simulink model "SC_Model_Sim_w3_final"  (R2023b)
settings: Solver=ode45  StartTime=0.0  StopTime=inf  FixedStep=0.001  RelTol=1e-3
values from neighbouring files (symbols this model uses):
  invJ = inv(J)    [SC_Model_Par.m]
  J = [J_11  0   0 ... (first row only)    [SC_Model_Par.m]
  J_w = wheel_momentum_max/wheel_speed_max    (= 0.000713699296376)    [SC_Model_Par.m]
  k_d = 0.2    [SC_Model_Par.m]
  k_p = 0.0041    [SC_Model_Par.m]
  mu_0 = 1.25663706212e-6    (= 1.25663706212e-06)    [SC_Model_Par.m]
  q_0 = dcm2quat(DCM_0)    [SC_Model_Par.m]
  R_E = 6371.2e3    (= 6371200)    [SC_Model_Par.m]
  wheel_momentum_max = 0.05    [SC_Model_Par.m]
  wheel_torque_max = 20e-3    (= 0.02)    [SC_Model_Par.m]
undefined symbols (not defined in the file or in its folder): IAU, juliandate, M, phi_n, theta_n, WMM2020
libraries: sharedtransform x3, vrlib x3, sharedutil x2, simulink x1, aerolibtransform2 x1, aerolibgravity2 x1
settings Model: SimulationMode=accelerator  Creator=andry  LastModifiedBy=Thien
settings SolverCC: ZeroCrossAlgorithm=Adaptive
settings DebuggingCC: MaskedZcDiagnostic=none  IgnoredZcDiagnostic=none  UnconnectedInputMsg=warning  UnconnectedOutputMsg=warning  UnconnectedLineMsg=warning
settings ModelReferenceCC: EnableRefExpFcnMdlSchedulingChecks=on
settings RTWCC: DLArmComputeVersion=19.05

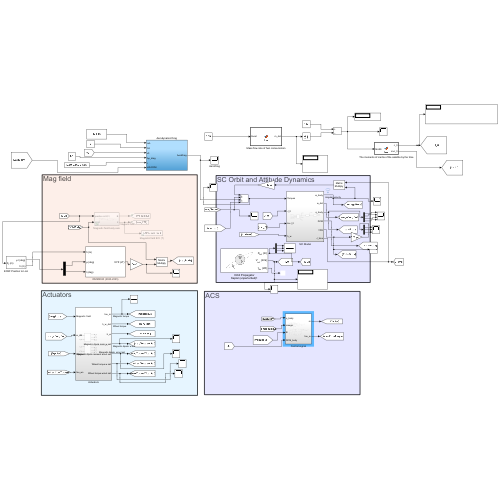
[thumbnail: Simulink's stored preview of the top-level diagram]
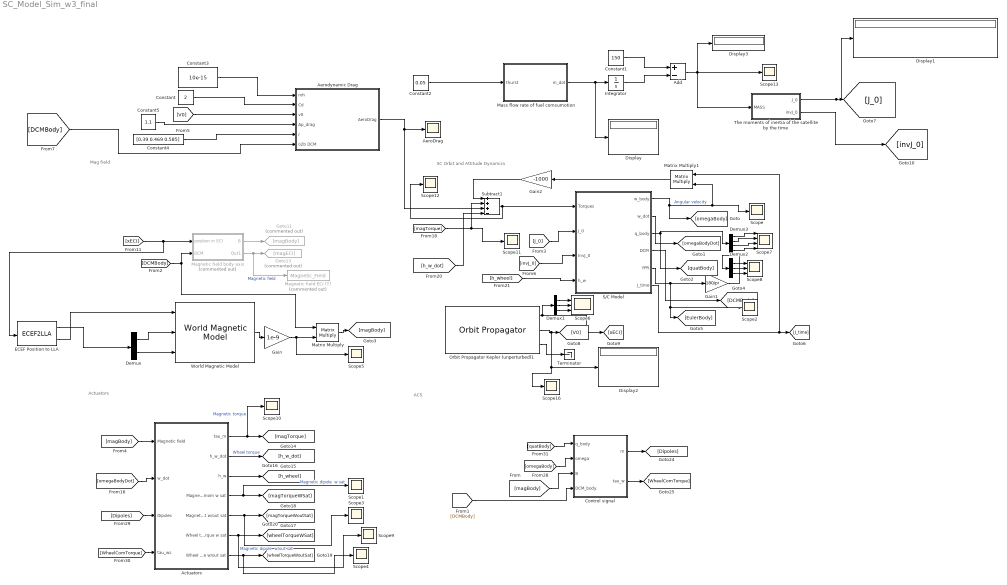
== system SC_Model_Sim_w3_final ==
  note: ACS
  note: Actuators
  note: SC Orbit and Attitude Dynamics
  note: Mag field
  Actuators : Subsystem
  Add : Sum  Inputs=+-
  AeroDrag : Scope
  Aerodynamic Drag : Subsystem
  Constant : Constant  Value=2
  Constant1 : Constant  Value=150  SampleTime=0
  Constant2 : Constant  Value=0.05  VectorParams1D=off
  Constant3 : Constant  Value=10e-15
  Constant4 : Constant  Value=[0.39 0.469 0.585]
  Constant5 : Constant  Value=1.1
  Control signal : Subsystem
  Demux : Demux  Outputs=2
  Demux1 : Demux  Outputs=3
  Demux2 : Demux  Outputs=3
  Demux3 : Demux
  Display{,1..3} (4 alike) : Display
      Display settings: Decimation=2
      Display1 settings: Decimation=3
  ECEF Position to LLA : ECEF2LLA
  Gain : Gain  Gain=1e-9
  Gain1 : Gain  Gain=180/pi
  Gain2 : Gain  Gain=-1000
  Goto11 : Goto  Commented=on  GotoTag=magBody
  Goto13 : Goto  Commented=on  GotoTag=magECI
  Integrator : Integrator  InitialCondition=35e-1000000  LimitOutput=on  UpperSaturationLimit=10  LowerSaturationLimit=0
  Magnetic field ECI (T) : ToWorkspace  Commented=on  VariableName=Magnetic_Field  SaveFormat=Timeseries  SampleTime=-1
  Magnetic field body axis : Subsystem  Commented=on
  Mass flow rate of fuel comsumotion : MATLAB Function  TreatAsAtomicUnit=on
  Matrix Multiply : Product  Multiplication=Matrix(*)
  Matrix Multiply1 : Product  Multiplication=Matrix(*)
  Orbit Propagator Kepler (unperturbed)1 : OrbitPropagator  outportFrame=Fixed-frame  startDate=juliandate(2022, 4, 25, 12, 0, 0)  semiMajorAxis=sma  eccentricity=ecc  inclination=orb_i  raan=RAAN  argPeriapsis=arg_per  trueAnomaly=0*pi/180  inertialPosition=[3649700.0 3308200.0 -4676600.0]  inertialVelocity=[-2750.8 6666.4 2573.4]  fixedPosition=[-4142689.0 -2676864.7 -4669861.6]  fixedVelocity=[1452.7 -6720.7 2568.1]  gravityModel=None  customR=3396200  customMu=4.305e13  customJ2=1.0826269e-03  customOmega=4.06125949e-3  useEOPs=off  angleUnits=Radians
  S/C Model : Subsystem
  Scope{,1..5,9..13,16} (12 alike) : Scope
  Scope6 : Scope  NumInputPorts=3
  Scope7 : Scope  NumInputPorts=4
  Scope8 : Scope  NumInputPorts=3
  Subtract1 : Sum  Inputs=+++-
  Terminator : Terminator
  The moments of inertia of the satellite by the time : MATLAB Function  TreatAsAtomicUnit=on
  World Magnetic Model : aerolibgravity2/World Magnetic Model  model=WMM2020 (2020-2025)  customFile='WMM2020.COF'  units=Metric (MKS)  time_in=off  month=April  day=25  year=2022  action=Error  h_out=off  dec_out=off  inc_out=off  ti_out=off
  wires:
  S/C Model/1(w_body) -> [omegaBody], Matrix Multiply1/2, Scope/1  "Angular velocity"
  S/C Model/2(w_dot) -> [omegaBodyDot]
  [DCMBody] -> Magnetic field body axis/2(DCM), Matrix Multiply/1
  S/C Model/5(YPR) -> [EulerBody], Scope2/1, Gain1/1
  [xECI] -> Magnetic field body axis/1(position in ECI), ECEF Position to LLA/1
  Orbit Propagator Kepler (unperturbed)1/2 -> Scope16/1, Display2/1, [V0]
  Magnetic field body axis/1(B) -> Goto11/1
  Magnetic field body axis/2(Out1) -> Magnetic field ECI (T)/1, Goto13/1  "Magnetic field"
  Actuators/1(tau_m) -> Scope10/1, [magTorque]  "Magnetic torque"
  Actuators/2(h_w_dot) -> [h_w_dot]  "Wheel torque"
  Actuators/3(h_w) -> [h_wheel]
  [h_wheel] -> S/C Model/4(h_w)
  Actuators/5(Magnetic dipole moment w/out sat) -> Scope3/1, [magTorqueWoutSat]  "Magnetic dipole  w/out sat"
  Actuators/4(Magnetic dipole mom w sat) -> Scope1/1, [magTorqueWSat]  "Magnetic dipole  w sat"
  Actuators/7(Wheel torque w/out sat) -> Scope4/1, [wheelTorqueWoutSat]
  Actuators/6(Wheel torque w sat) -> Scope9/1, [wheelTorqueWSat]
  [magBody] -> Actuators/1(Magnetic field)
  [omegaBodyDot] -> Actuators/2(w_dot)
  Control signal/1(m) -> [Dipoles]
  Control signal/2(tau_w) -> [WheelComTorque]
  [Dipoles] -> Actuators/3(Dipoles)
  [WheelComTorque] -> Actuators/4(tau_ws)
  Orbit Propagator Kepler (unperturbed)1/3 -> Terminator/1
  [quatBody] -> Control signal/1(q_body)
  [omegaBody] -> Control signal/2(omega)
  [magBody] -> Control signal/3(B)
  ECEF Position to LLA/2 -> World Magnetic Model/1
  ECEF Position to LLA/1 -> Demux/1
  Demux/1 -> World Magnetic Model/2
  Demux/2 -> World Magnetic Model/3
  World Magnetic Model/1 -> Gain/1
  Matrix Multiply/1 -> [magBody]
  Demux1/1 -> Scope6/1
  Demux1/2 -> Scope6/2
  Demux1/3 -> Scope6/3
  Orbit Propagator Kepler (unperturbed)1/1 -> Demux1/1, [xECI]
  Gain/1 -> Scope5/1, Matrix Multiply/2
  S/C Model/3(q_body) -> Demux3/1, [quatBody]
  Demux2/1 -> Scope8/1
  Demux2/2 -> Scope8/2
  Demux2/3 -> Scope8/3
  Gain1/1 -> Demux2/1
  Demux3/1 -> Scope7/1
  Demux3/2 -> Scope7/2
  Demux3/3 -> Scope7/3
  Demux3/4 -> Scope7/4
  [magTorque] -> Scope11/1, Subtract1/2
  Gain2/1 -> Subtract1/1
  Subtract1/1 -> Scope12/1, S/C Model/1(Torques)
  The moments of inertia of the satellite by the time/1(J_0) -> Display1/1, [J_0]
  [V0] -> Aerodynamic Drag/3(v0)
  Constant/1 -> Aerodynamic Drag/2(Cd)
  [J_0] -> S/C Model/2(J_0)
  The moments of inertia of the satellite by the time/2(invJ_0) -> [invJ_0]
  [invJ_0] -> S/C Model/3(InvJ_0)
  Matrix Multiply1/1 -> Gain2/1
  S/C Model/6(J_time) -> [J_time], Matrix Multiply1/1
  Constant2/1 -> Mass flow rate of fuel comsumotion/1(thurst)
  Mass flow rate of fuel comsumotion/1(m_dot) -> Display/1, Integrator/1
  Add/1 -> The moments of inertia of the satellite by the time/1(MASS), Scope13/1, Display3/1
  Integrator/1 -> Add/2
  Constant1/1 -> Add/1
  [DCMBody] -> Control signal/4(DCM_body)
  Constant3/1 -> Aerodynamic Drag/1(roh)
  Constant4/1 -> Aerodynamic Drag/5(r)
  Constant5/1 -> Aerodynamic Drag/4(Ap_drag)
  S/C Model/4(DCM) -> [DCMBody]
  [h_w_dot] -> Subtract1/4
  Aerodynamic Drag/1(AeroDrag) -> Subtract1/3, AeroDrag/1
  [DCMBody] -> Aerodynamic Drag/6(o2b DCM)

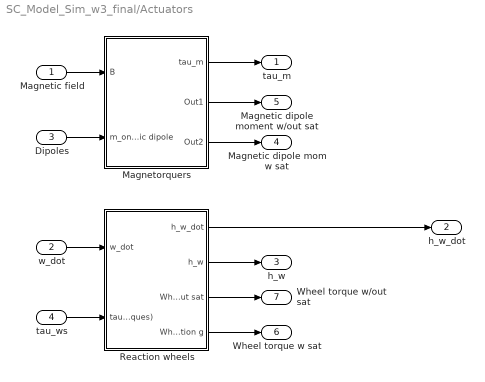
== system SC_Model_Sim_w3_final/Actuators ==
  Magnetic field : Inport
  w_dot : Inport  Port=2
  Dipoles : Inport  Port=3
  tau_ws : Inport  Port=4
  Magnetorquers : Subsystem
  Reaction wheels : Subsystem
  tau_m : Outport
  h_w_dot : Outport  Port=2
  h_w : Outport  Port=3
  Magnetic dipole mom w sat : Outport  Port=4
  Magnetic dipole moment w/out sat : Outport  Port=5
  Wheel torque w sat : Outport  Port=6
  Wheel torque w/out sat : Outport  Port=7
  wires:
  w_dot/1 -> Reaction wheels/1(w_dot)
  Reaction wheels/1(h_w_dot) -> h_w_dot/1
  Reaction wheels/2(h_w) -> h_w/1
  Magnetorquers/2(Out1) -> Magnetic dipole moment w/out sat/1
  Magnetorquers/3(Out2) -> Magnetic dipole mom w sat/1
  Reaction wheels/4(Wheel torque w saturation g) -> Wheel torque w sat/1
  Reaction wheels/3(Wheel torque w/out sat) -> Wheel torque w/out sat/1
  Dipoles/1 -> Magnetorquers/2(m_onboard magnetic dipole)
  Magnetic field/1 -> Magnetorquers/1(B)
  tau_ws/1 -> Reaction wheels/2(tau_w (control torques))
  Magnetorquers/1(tau_m) -> tau_m/1

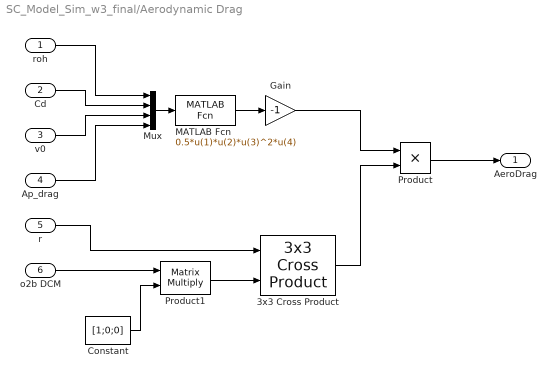
== system SC_Model_Sim_w3_final/Aerodynamic Drag ==
  roh : Inport
  Cd : Inport  Port=2
  v0 : Inport  Port=3
  Ap_drag : Inport  Port=4
  r : Inport  Port=5
  o2b DCM : Inport  Port=6
  3x3 Cross Product : sharedutil/3x3 Cross Product  aMode=aMode
      settings: LibrarySourceBlock=aerolibutil/3x3 Cross Product
  Constant : Constant  Value=[1;0;0]
  Gain : Gain  Gain=-1
  MATLAB Fcn : MATLABFcn  MATLABFcn=0.5*u(1)*u(2)*u(3)^2*u(4)
  Mux : Mux
  Product : Product  RndMeth=Zero
  Product1 : Product  Multiplication=Matrix(*)  RndMeth=Zero
  AeroDrag : Outport
  wires:
  Mux/1 -> MATLAB Fcn/1
  roh/1 -> Mux/1
  Cd/1 -> Mux/2
  v0/1 -> Mux/3
  Ap_drag/1 -> Mux/4
  Constant/1 -> Product1/2
  o2b DCM/1 -> Product1/1
  Product1/1 -> 3x3 Cross Product/2
  r/1 -> 3x3 Cross Product/1
  MATLAB Fcn/1 -> Gain/1
  Gain/1 -> Product/1
  3x3 Cross Product/1 -> Product/2
  Product/1 -> AeroDrag/1

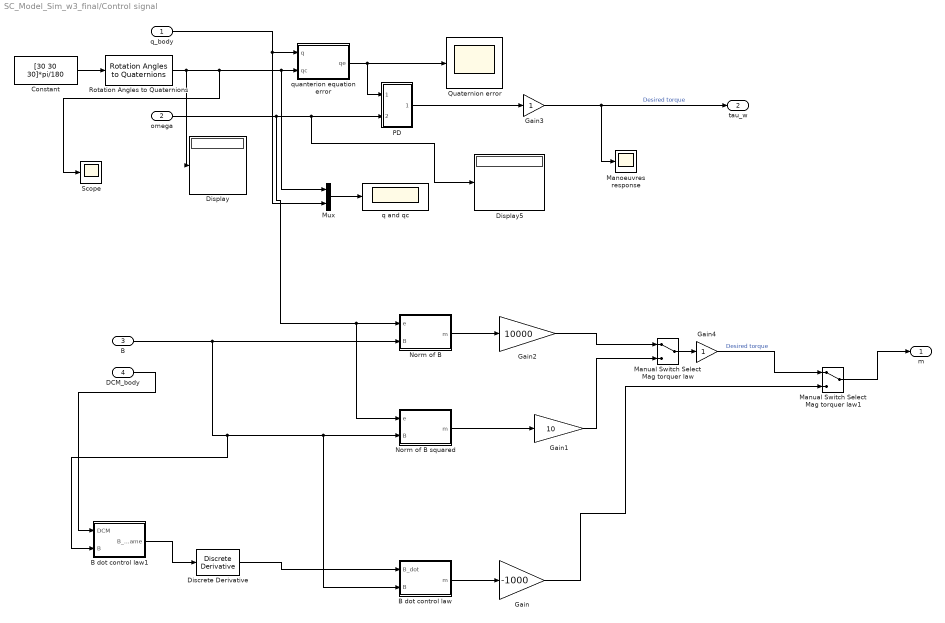
== system SC_Model_Sim_w3_final/Control signal ==
  q_body : Inport
  omega : Inport  Port=2
  B : Inport  Port=3
  DCM_body : Inport  Port=4
  B dot control law : MATLAB Function  TreatAsAtomicUnit=on
  B dot control law1 : MATLAB Function  TreatAsAtomicUnit=on
  Constant : Constant  Value=[30 30 30]*pi/180  VectorParams1D=off
  Discrete Derivative : simulink/Discrete/Discrete Derivative  gainval=1.0  ICPrevScaledInput=0.0  OutMin=[]  OutMax=[]  OutDataType=fixdt(1, 16)  OutScaling=2^-10  DoSatur=off
  Display : Display
  Display5 : Display
  Gain : Gain  Gain=-1000
  Gain1 : Gain  Gain=10
  Gain2 : Gain  Gain=10000
  Gain3 : Gain
  Gain4 : Gain
  Manoeuvres response : Scope
  Manual Switch Select Mag torquer law : ManualSwitch
  Manual Switch Select Mag torquer law1 : ManualSwitch
  Mux : Mux  Inputs=2
  Norm of B : MATLAB Function  TreatAsAtomicUnit=on
  "Norm of B squared " : MATLAB Function  TreatAsAtomicUnit=on
  PD : Subsystem
  Quaternion error : Scope
  Rotation Angles to Quaternions : sharedtransform/Rotation Angles to Quaternions  rotationOrder=ZYX  aMode=aMode
  Scope : Scope
  q and qc : Scope
  quanterion equation error : MATLAB Function  TreatAsAtomicUnit=on
  m : Outport
  tau_w : Outport  Port=2
  wires:
  PD/1(tau) -> Gain3/1
  Gain3/1 -> tau_w/1, Manoeuvres response/1  "Desired torque"
  omega/1 -> "Norm of B squared "/1(e), Norm of B/1(e), Display5/1, PD/2(w_body)
  Manual Switch Select Mag torquer law/1 -> Gain4/1
  Norm of B/1(m) -> Gain2/1
  Gain1/1 -> Manual Switch Select Mag torquer law/2
  "Norm of B squared "/1(m) -> Gain1/1
  Constant/1 -> Rotation Angles to Quaternions/1
  quanterion equation error/1(qe) -> PD/1(q_body), Quaternion error/1
  q_body/1 -> Mux/2, quanterion equation error/1(q)
  Mux/1 -> q and qc/1
  Rotation Angles to Quaternions/1 -> Scope/1, Mux/1, quanterion equation error/2(qc), Display/1
  B/1 -> B dot control law1/2(B), B dot control law/2(B), "Norm of B squared "/2(B), Norm of B/2(B)
  Gain2/1 -> Manual Switch Select Mag torquer law/1
  B dot control law/1(m) -> Gain/1
  Gain/1 -> Manual Switch Select Mag torquer law1/2
  Discrete Derivative/1 -> B dot control law/1(B_dot)
  Gain4/1 -> Manual Switch Select Mag torquer law1/1  "Desired torque"
  Manual Switch Select Mag torquer law1/1 -> m/1
  B dot control law1/1(B_bodyframe) -> Discrete Derivative/1
  DCM_body/1 -> B dot control law1/1(DCM)

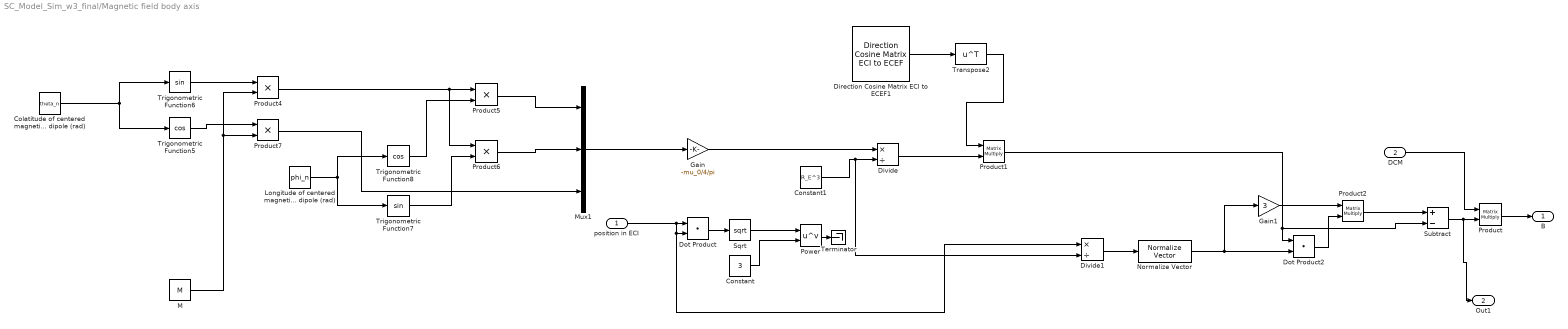
== system SC_Model_Sim_w3_final/Magnetic field body axis ==
  position in ECI : Inport
  DCM : Inport  Port=2
  Colatitude of centered magnetic dipole (rad) : Constant  Value=theta_n
  Constant : Constant  Value=3
  Constant1 : Constant  Value=R_E^3
  Direction Cosine Matrix ECI to ECEF1 : aerolibtransform2/Direction Cosine Matrix ECI to ECEF  red=IAU-2000/2006  year=2020  month=January  day=1  hour=0  min=0  sec=0  deltaT=None  errorflag=Error  extraparamflag=off
      settings: AttributesFormatString=%<red>
  Divide : Product  Inputs=*/
  Divide1 : Product  Inputs=*/
  Dot Product : DotProduct  OutDataTypeStr=Inherit: Inherit via internal rule
  Dot Product2 : DotProduct  OutDataTypeStr=Inherit: Inherit via internal rule
  Gain : Gain  Gain=-mu_0/4/pi
  Gain1 : Gain  Gain=3
  Longitude of centered magnetic dipole (rad) : Constant  Value=phi_n
  M : Constant  Value=M
  Mux1 : Mux  Inputs=3
  Normalize Vector : vrlib/Utilities/Normalize Vector  maxzero=0
  Power : Math  Operator=pow
  Product : Product  Multiplication=Matrix(*)
  Product1 : Product  Multiplication=Matrix(*)
  Product2 : Product  Multiplication=Matrix(*)
  Product{4..7} (4 alike) : Product
  Sqrt : Sqrt
  Subtract : Sum  Inputs=+-
  Terminator : Terminator
  Transpose2 : Math  Operator=transpose  SignedPower=on  RndMeth=Zero
  Trigonometric Function5 : Trigonometry  Operator=cos
  Trigonometric Function6 : Trigonometry
  Trigonometric Function7 : Trigonometry
  Trigonometric Function8 : Trigonometry  Operator=cos
  B : Outport
  Out1 : Outport  Port=2
  wires:
  Longitude of centered magnetic dipole (rad)/1 -> Trigonometric Function7/1, Trigonometric Function8/1
  Product4/1 -> Product6/1, Product5/1
  Product6/1 -> Mux1/2
  M/1 -> Product7/2, Product4/2
  Colatitude of centered magnetic dipole (rad)/1 -> Trigonometric Function5/1, Trigonometric Function6/1
  Trigonometric Function7/1 -> Product6/2
  Trigonometric Function6/1 -> Product4/1
  Product7/1 -> Mux1/3
  Trigonometric Function8/1 -> Product5/2
  Product5/1 -> Mux1/1
  Trigonometric Function5/1 -> Product7/1
  Mux1/1 -> Gain/1
  Dot Product/1 -> Sqrt/1
  Constant/1 -> Power/2
  Sqrt/1 -> Power/1
  Gain/1 -> Divide/1
  Divide/1 -> Product1/2
  Direction Cosine Matrix ECI to ECEF1/1 -> Transpose2/1
  Transpose2/1 -> Product1/1
  Subtract/1 -> Out1/1, Product/2
  Dot Product2/1 -> Product2/2
  Gain1/1 -> Product2/1
  Product2/1 -> Subtract/1
  position in ECI/1 -> Dot Product/2, Divide1/1, Dot Product/1
  Product1/1 -> Subtract/2, Dot Product2/1
  DCM/1 -> Product/1
  Product/1 -> B/1
  Constant1/1 -> Divide/2, Divide1/2
  Divide1/1 -> Normalize Vector/1
  Normalize Vector/1 -> Gain1/1, Dot Product2/2
  Power/1 -> Terminator/1

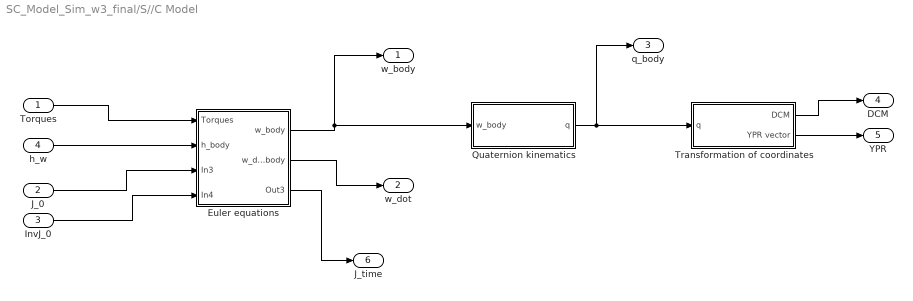
== system SC_Model_Sim_w3_final/S//C Model ==
  Torques : Inport
  J_0 : Inport  Port=2
  InvJ_0 : Inport  Port=3
  h_w : Inport  Port=4
  Euler equations : Subsystem
  Quaternion kinematics : Subsystem
  Transformation of coordinates : Subsystem
  w_body : Outport
  w_dot : Outport  Port=2
  q_body : Outport  Port=3
  DCM : Outport  Port=4
  YPR : Outport  Port=5
  J_time : Outport  Port=6
  wires:
  Quaternion kinematics/1(q) -> q_body/1, Transformation of coordinates/1(q)
  Transformation of coordinates/2(YPR vector) -> YPR/1
  Euler equations/2(w_dot_body) -> w_dot/1
  h_w/1 -> Euler equations/2(h_body)
  Transformation of coordinates/1(DCM) -> DCM/1
  Euler equations/1(w_body) -> w_body/1, Quaternion kinematics/1(w_body)
  Torques/1 -> Euler equations/1(Torques)
  J_0/1 -> Euler equations/3(In3)
  InvJ_0/1 -> Euler equations/4(In4)
  Euler equations/3(Out3) -> J_time/1

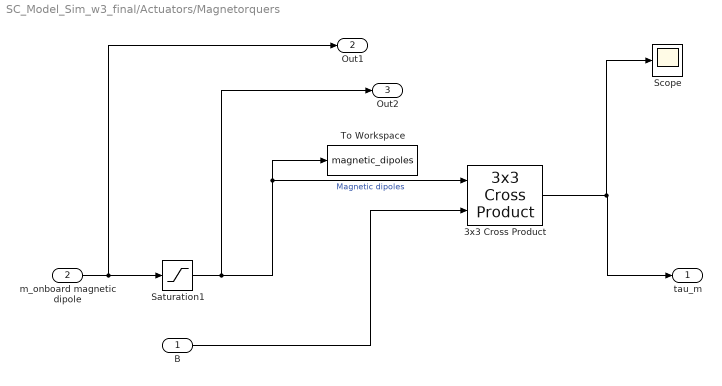
== system SC_Model_Sim_w3_final/Actuators/Magnetorquers ==
  B : Inport
  m_onboard magnetic dipole : Inport  Port=2
  3x3 Cross Product : sharedutil/3x3 Cross Product  aMode=aMode
  Saturation1 : Saturate  UpperLimit=20  LowerLimit=-20
  Scope : Scope
  To Workspace : ToWorkspace  VariableName=magnetic_dipoles  SaveFormat=Timeseries  SampleTime=-1
  tau_m : Outport
  Out1 : Outport  Port=2
  Out2 : Outport  Port=3
  wires:
  B/1 -> 3x3 Cross Product/2
  3x3 Cross Product/1 -> Scope/1, tau_m/1
  Saturation1/1 -> Out2/1, 3x3 Cross Product/1, To Workspace/1  "Magnetic dipoles"
  m_onboard magnetic dipole/1 -> Out1/1, Saturation1/1

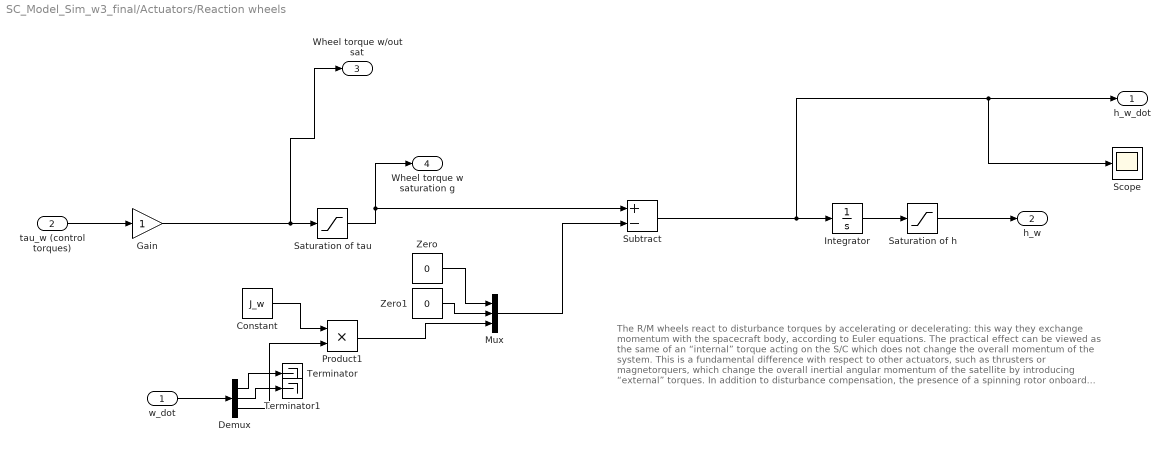
== system SC_Model_Sim_w3_final/Actuators/Reaction wheels ==
  note: The R/M wheels react to disturbance torques by accelerating or decelerating: this way they exchange momentum with the
      | spacecraft body, according to Euler equations. The practical effect can be viewed as the same of an “internal” torque acting
      | on the S/C which does not change the overall momentum of the system. This is a fundamental difference with respect to
      | other actuators, such as thrusters or magnetorquers, which change the overall inertial angular momentum of the satellite by
      | introducing “external” torques.
      | In addition to disturbance compensation, the presence of a spinning rotor onboard generates a gyroscopic stiffness
      | (i.e. storage of angular momentum) making the S/C less sensitive to the disturbance torques. Depending on which of the two
      | features above, reaction to disturbance or storage of momentum, is given the priority, a distinction is made between reaction wheels (RW)
      | or momentum wheels (MW).
      | A MW is used to keep the actuation axis almost inertially fixed by rotating at a nominal rate different
      | from zero; a control of the attitude about the rotation axis is allowed by variation of the wheel speed.
      | Conversely, RWs have zero nominal speed.
  w_dot : Inport
  tau_w (control torques) : Inport  Port=2
  Constant : Constant  Value=J_w
  Demux : Demux  Outputs=3
  Gain : Gain
  Integrator : Integrator
  Mux : Mux  Inputs=3
  Product1 : Product
  Saturation of h : Saturate  UpperLimit=wheel_momentum_max*100  LowerLimit=-wheel_momentum_max*100
  Saturation of tau : Saturate  UpperLimit=wheel_torque_max  LowerLimit=-wheel_torque_max
  Scope : Scope
  Subtract : Sum  Inputs=+-
  Terminator : Terminator
  Terminator1 : Terminator
  Zero : Constant  Value=0  OutDataTypeStr=Inherit: Inherit via back propagation
  Zero1 : Constant  Value=0  OutDataTypeStr=Inherit: Inherit via back propagation
  h_w_dot : Outport
  h_w : Outport  Port=2
  Wheel torque w/out sat : Outport  Port=3
  Wheel torque w saturation g : Outport  Port=4
  wires:
  Constant/1 -> Product1/1
  w_dot/1 -> Demux/1
  Demux/1 -> Terminator/1
  Zero/1 -> Mux/1
  Mux/1 -> Subtract/2
  Integrator/1 -> Saturation of h/1
  Saturation of tau/1 -> Wheel torque w saturation g/1, Subtract/1
  Saturation of h/1 -> h_w/1
  tau_w (control torques)/1 -> Gain/1
  Subtract/1 -> Scope/1, h_w_dot/1, Integrator/1
  Demux/2 -> Terminator1/1
  Demux/3 -> Product1/2
  Gain/1 -> Wheel torque w/out sat/1, Saturation of tau/1
  Zero1/1 -> Mux/2
  Product1/1 -> Mux/3

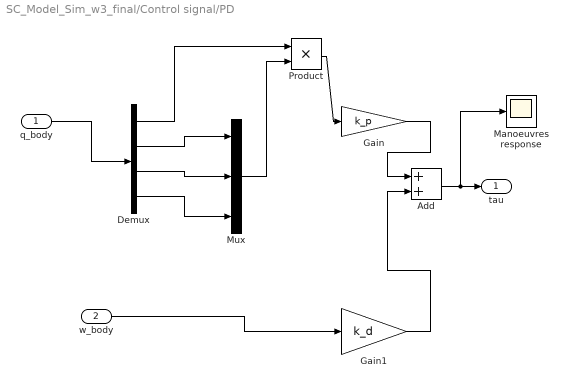
== system SC_Model_Sim_w3_final/Control signal/PD ==
  q_body : Inport
  w_body : Inport  Port=2
  Add : Sum
  Demux : Demux
  Gain : Gain  Gain=k_p
  Gain1 : Gain  Gain=k_d
  Manoeuvres response : Scope
  Mux : Mux  Inputs=3
  Product : Product
  tau : Outport
  wires:
  Gain1/1 -> Add/2
  Demux/1 -> Product/1
  q_body/1 -> Demux/1
  Add/1 -> Manoeuvres response/1, tau/1
  w_body/1 -> Gain1/1
  Demux/2 -> Mux/1
  Demux/3 -> Mux/2
  Demux/4 -> Mux/3
  Mux/1 -> Product/2
  Product/1 -> Gain/1
  Gain/1 -> Add/1

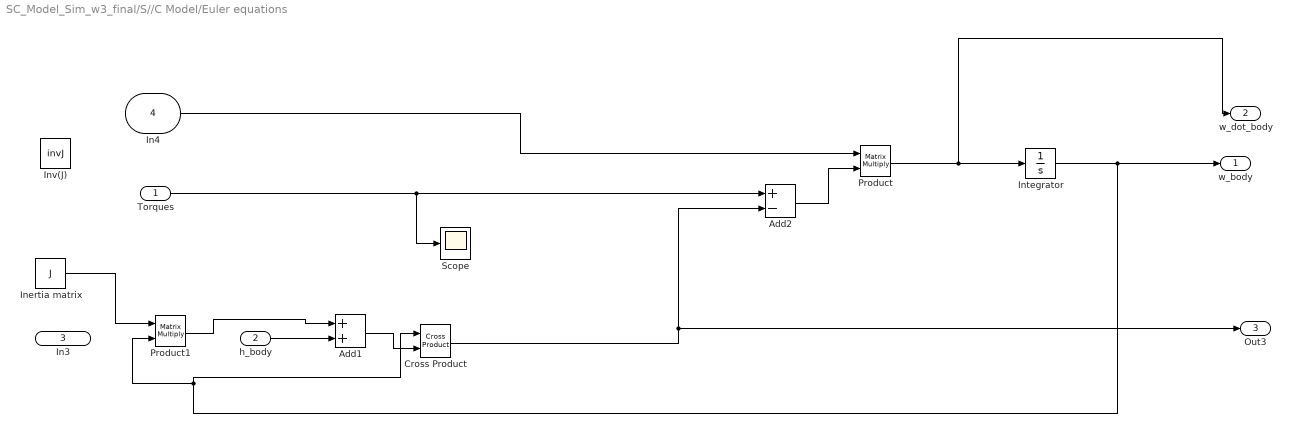
== system SC_Model_Sim_w3_final/S//C Model/Euler equations ==
  Torques : Inport
  h_body : Inport  Port=2
  In3 : Inport  Port=3
  In4 : Inport  Port=4
  Add1 : Sum
  Add2 : Sum  Inputs=+-
  Cross Product : vrlib/Utilities/Cross Product
  Inertia matrix : Constant  Value=J
  Integrator : Integrator  InitialCondition=[0.2 0.2 0.2]
  Inv(J) : Constant  Value=invJ
  Product : Product  Multiplication=Matrix(*)
  Product1 : Product  Multiplication=Matrix(*)
  Scope : Scope
  w_body : Outport
  w_dot_body : Outport  Port=2
  Out3 : Outport  Port=3
  wires:
  Add1/1 -> Cross Product/2
  Product1/1 -> Add1/1
  Add2/1 -> Product/2
  Torques/1 -> Add2/1, Scope/1
  h_body/1 -> Add1/2
  Integrator/1 -> w_body/1, Cross Product/1, Product1/2
  Product/1 -> w_dot_body/1, Integrator/1
  Cross Product/1 -> Add2/2, Out3/1
  Inertia matrix/1 -> Product1/1
  In4/1 -> Product/1

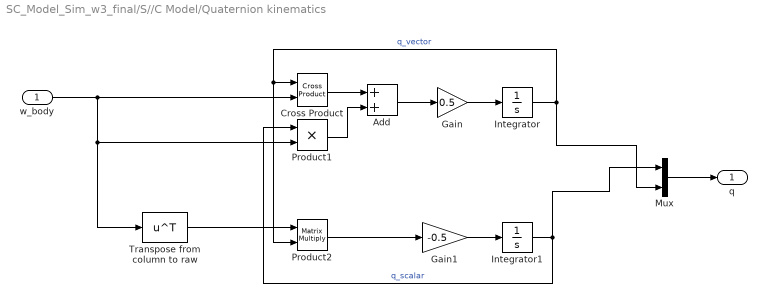
== system SC_Model_Sim_w3_final/S//C Model/Quaternion kinematics ==
  w_body : Inport
  Add : Sum
  Cross Product : vrlib/Utilities/Cross Product
  Gain : Gain  Gain=0.5
  Gain1 : Gain  Gain=-0.5
  Integrator : Integrator  InitialCondition=q_0(2:4)
  Integrator1 : Integrator  InitialCondition=q_0(1)
  Mux : Mux  Inputs=2
  Product1 : Product
  Product2 : Product  Multiplication=Matrix(*)
  Transpose from column to raw : Math  Operator=transpose  SignedPower=on  RndMeth=Zero
  q : Outport
  wires:
  Gain/1 -> Integrator/1
  w_body/1 -> Cross Product/2, Transpose from column to raw/1, Product1/2
  Cross Product/1 -> Add/1
  Product1/1 -> Add/2
  Add/1 -> Gain/1
  Integrator/1 -> Mux/2, Product2/2, Cross Product/1  "q_vector"
  Transpose from column to raw/1 -> Product2/1
  Product2/1 -> Gain1/1
  Gain1/1 -> Integrator1/1
  Integrator1/1 -> Mux/1, Product1/1  "q_scalar"
  Mux/1 -> q/1

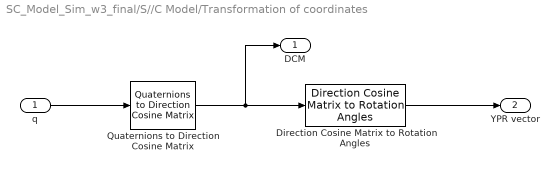
== system SC_Model_Sim_w3_final/S//C Model/Transformation of coordinates ==
  q : Inport
  Direction Cosine Matrix to Rotation Angles : sharedtransform/Direction Cosine Matrix to Rotation Angles  rotationOrder=ZYX  aMode=aMode  action=None  tolerance=eps(2)
  Quaternions to Direction Cosine Matrix : sharedtransform/Quaternions to  Direction Cosine Matrix  aMode=aMode
  DCM : Outport
  YPR vector : Outport  Port=2
  wires:
  q/1 -> Quaternions to Direction Cosine Matrix/1
  Quaternions to Direction Cosine Matrix/1 -> DCM/1, Direction Cosine Matrix to Rotation Angles/1
  Direction Cosine Matrix to Rotation Angles/1 -> YPR vector/1

== matlab function SC_Model_Sim_w3_final/Control signal/Norm of B squared  ==
  data: e input; m output; B input
function m = fcn(e,B)

m = cross(e,B)/(norm(B)^2);

== matlab function SC_Model_Sim_w3_final/Control signal/Norm of B ==
  data: e input; m output; B input
function m = fcn(e,B)

m = cross(e,B)/(norm(B));

== matlab function SC_Model_Sim_w3_final/Control signal/quanterion equation error ==
  data: q input; qe output; qc input
function qe = fcn(q,qc)

qe1 = qc(1)*q(2)+qc(4)*q(3)-qc(3)*q(4)-qc(2)*q(1);
qe2 = -qc(4)*q(2)+qc(1)*q(3)+qc(2)*q(4)-qc(3)*q(1);
qe3 = qc(3)*q(2)-qc(2)*q(3)+qc(1)*q(4)-qc(4)*q(1);
qe0 = qc(2)*q(2)+qc(3)*q(3)+qc(4)*q(4) + qc(1)*q(1);

qe=[qe0;qe1;qe2;qe3];

== matlab function SC_Model_Sim_w3_final/Mass flow rate of fuel comsumotion ==
  data: m_dot output; thurst input
function m_dot  = fcn(thurst)


dim_1=0.724/2;                                                   % Dimension 1 [m]
dim_2=0.696/2;                                                    % Dimension 2 [m]
dim_3=1.018/2;                                                    % Dimension 3 [m]

a = [dim_1 dim_2 dim_3];

b = norm(a);
g0 = 9.81;

m_dot = (thurst)/(b*g0*200);

== matlab function SC_Model_Sim_w3_final/Control signal/B dot control law ==
  data: B_dot input; m output; B input
function m = fcn(B_dot,B)

m = B_dot/(norm(B)^2);

== matlab function SC_Model_Sim_w3_final/Control signal/B dot control law1 ==
  data: DCM input; B_bodyframe output; B input
function B_bodyframe  = fcn(DCM,B)

a = norm(DCM);
B_bodyframe = a .* B;

== matlab function SC_Model_Sim_w3_final/The moments of inertia of the satellite by the time ==
  data: MASS input; J_0 output; invJ_0 output
function [J_0,invJ_0]   = fcn(MASS)

dim_1=0.696;                                                   % Dimension 1 [m]
dim_2=0.724;                                                   % Dimension 2 [m]
dim_3=1.018;                                                    % Dimension 3 [m]


sat_mass = MASS;                                                   % Mass[Kg]

J_44=sat_mass/12*(dim_2^2+dim_3^2);                           % Moment of inertia along 1 [Kg*m^2]
J_55=sat_mass/12*(dim_1^2+dim_3^2);                           % Moment of inertia along 2 [Kg*m^2]
J_66=sat_mass/12*(dim_1^2+dim_2^2);                           % Moment of inertia along 3 [Kg*m^2]



J_0 = [J_44  0   0                                              % Matrix of inertia
       0  J_55   0
       0  0   J_66];

invJ_0 = inv(J_0);
